simulink model "prob4"  (R2020b)
settings: Solver=VariableStepAuto  StartTime=0.0  StopTime=10.0  RelTol=1e-3
values from neighbouring files (symbols this model uses):
  b = 0.1    [motor_control_model_variables.sldd]    (also in variable_values.mat; variables.mat = 3.5077e-06)
  J = 0.01    [motor_control_model_variables.sldd]    (also in variable_values.mat; variables.mat = 3.2284e-06)
  K = 0.01    [motor_control_model_variables.sldd]    (also in variable_values.mat; variables.mat = 0.0274)
  L = 2.75E-6    [motor_control_model_variables.sldd]    (also in variable_values.mat = 0.5; variables.mat = 2.75e-06)
  R = 4.0    [motor_control_model_variables.sldd]    (also in variable_values.mat = 1; variables.mat = 4)
settings Model: Creator=DELL  LastModifiedBy=DELL

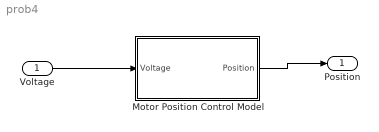
== system prob4 ==
  Voltage : Inport  OutDataTypeStr=double  PortDimensions=1  SampleTime=0
  Motor Position Control Model : Subsystem
  Position : Outport  OutDataTypeStr=double  PortDimensions=1  SampleTime=0
  wires:
  Voltage/1 -> Motor Position Control Model/1(Voltage)
  Motor Position Control Model/1(Position) -> Position/1

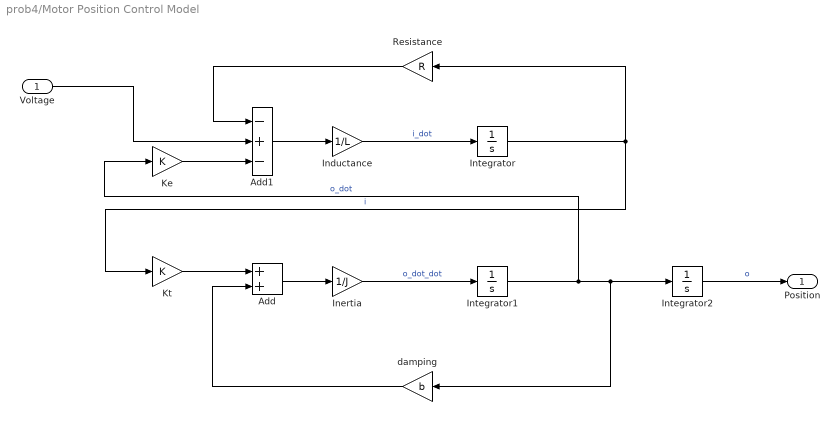
== system prob4/Motor Position Control Model ==
  Voltage : Inport  OutDataTypeStr=double  PortDimensions=1  SampleTime=0
  Add : Sum
  Add1 : Sum  Inputs=-+-
  Inductance : Gain  Gain=1/L
  Inertia : Gain  Gain=1/J
  Integrator : Integrator
  Integrator1 : Integrator
  Integrator2 : Integrator
  Ke : Gain  Gain=K
  Kt : Gain  Gain=K
  Resistance : Gain  Gain=R
  damping : Gain  Gain=b
  Position : Outport  OutDataTypeStr=double  PortDimensions=1  SampleTime=0
  wires:
  Ke/1 -> Add1/3
  Integrator/1 -> Kt/1, Resistance/1  "i"
  Add1/1 -> Inductance/1
  Resistance/1 -> Add1/1
  Integrator1/1 -> Ke/1, damping/1, Integrator2/1  "o_dot"
  Voltage/1 -> Add1/2
  Inertia/1 -> Integrator1/1  "o_dot_dot"
  Inductance/1 -> Integrator/1  "i_dot"
  damping/1 -> Add/2
  Kt/1 -> Add/1
  Integrator2/1 -> Position/1  "o"
  Add/1 -> Inertia/1
